simulink model "OberverForPMSM"  (R2018b)
settings: Solver=FixedStepAuto  StartTime=0.0  StopTime=inf  FixedStep=Ts  MaxStep=Ts  RelTol=1e-3  EnableMultiTasking=on
PreLoadFcn:
  | Ts=1e-6;
  | deci=20;
InitFcn:
  | Ts=5e-6;
  | deci=20;
undefined symbols (not defined in the file or in its folder): DiscIntNeverNeededParam, level
libraries: powerlib_extras x37, powerlib x18, powerlib_meascontrol x8, simulink x5, simulink_extras x4
(part 1 of 2)
Description:
  | Copyright 2013-2015 Ruan Jiayang, Tsinghua Univ.
settings Model: SimulationMode=accelerator  Creator=XiaoLei  LastModifiedBy=Administrator
settings SolverCC: AlgebraicLoopSolver=LineSearch  AutoInsertRateTranBlk=on
settings DataIOCC: InitialState=xInit  LimitDataPoints=on  SaveFinalState=on  SaveFormat=StructureWithTime  SignalLoggingSaveFormat=ModelDataLogs  SaveOutput=off  SignalLogging=off  SaveTime=off
settings OptimizationCC: ExpressionDepthLimit=2147483647  InitFltsAndDblsToZero=on  LifeSpan=inf
settings DebuggingCC: SaveWithParameterizedLinksMsg=none  UnderspecifiedInitializationDetection=Classic  MergeDetectMultiDrivingBlocksExec=none  SignalResolutionControl=TryResolveAllWithWarning  SolverPrmCheckMsg=warning  MultiTaskDSMMsg=warning  MultiTaskCondExecSysMsg=none  FcnCallInpInsideContextMsg=warning  UnconnectedInputMsg=none  UnconnectedOutputMsg=none  UnconnectedLineMsg=none  StateNameClashWarn=warning  SFUnexpectedBacktrackingDiag=warning  SFNoUnconditionalDefaultTransitionDiag=warning  SFExecutionAtInitializationDiag=none
settings HardwareCC: ProdBitPerPointer=32  ProdBitPerSizeT=32  ProdBitPerPtrDiffT=32  ProdLargestAtomicFloat=None  ProdIntDivRoundTo=Undefined  ProdEndianess=Unspecified  ProdWordSize=32  ProdHWDeviceType=32-bit Generic
settings ModelReferenceCC: PropagateSignalLabelsOutOfModel=off
settings SFSimCC: SimUseLocalCustomCode=off  SimParseCustomCode=off
settings RTWCC: RTWUseLocalCustomCode=off
settings CodeAppCC: StateflowObjectComments=on
settings GRTTargetCC: TargetFcnLib=ansi_tfl_tmw.mat  TargetLangStandard=C89/C90 (ANSI)  GeneratePreprocessorConditionals=Disable all  CombineOutputUpdateFcns=off  GRTInterface=on
settings ConfigComp: CovMetricSettings=dw  CovHtmlReporting=on  CovSaveCumulativeToWorkspaceVar=on  CovSaveSingleToWorkspaceVar=on  CovExternalEMLEnable=off

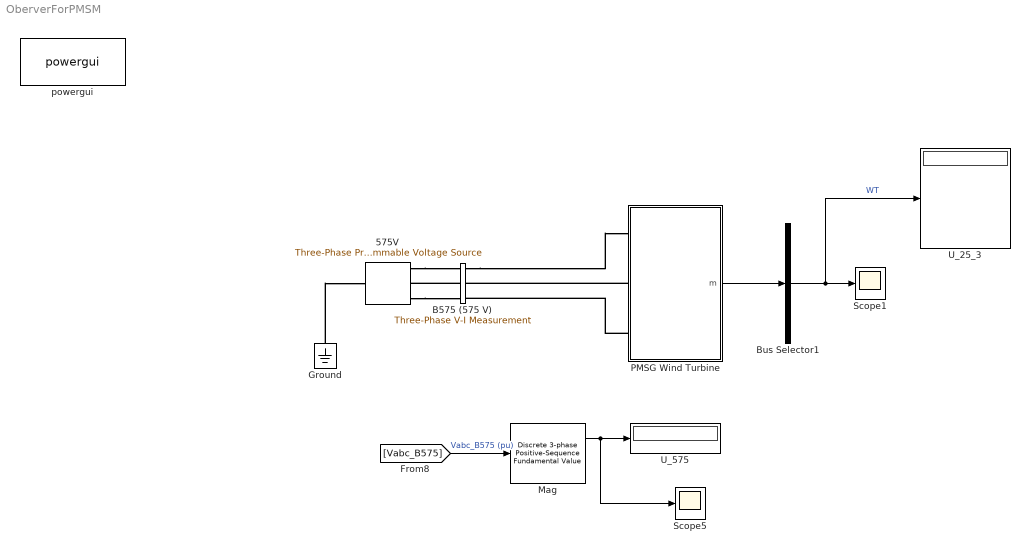
== system OberverForPMSM ==
  575V : powerlib/Electrical Sources/Three-Phase Programmable Voltage Source  PositiveSequence=[575 0 60]  VariationEntity=Amplitude  VariationType=Table of time-amplitude pairs  VariationTypeAlt=Step  VariationStep=-0.2  VariationRate=10  VariationMagnitude=0.3  VariationFrequency=2  VariationTiming=[0.05 0.05+5/60]  VariationPhaseA=off  Amplitudes=[1 0.5 1]  TimeValues=[0 20 20.3]  HarmonicGeneration=off  HarmonicA=[1 -0.1 0 2]  HarmonicB=[2 0.15 35 2]*0  Timing="[0.1  2]"  BusType=swing  Pref=0  Qref=0  Qmin=-inf  Qmax=inf
  B575 (575 V) : powerlib/Measurements/Three-Phase V-I Measurement  VoltageMeasurement=phase-to-ground  SetLabelV=on  LabelV=Vabc_B575  Vpu=on  VpuLL=off  CurrentMeasurement=yes  SetLabelI=on  LabelI=Iabc_B575  Ipu=on  Pbase=1.5e6  Vbase=575  OutputType=Complex  PhasorSimulation=off  PSBequivalent=0
  Bus Selector1 : BusSelector  OutputSignals=wr,Tem,Tm,PQ.P_pu,PQ.Q_pu  OutputAsBus=on
  Ground : powerlib/Elements/Ground  LConnTagsString=a
  Mag : powerlib_extras/Discrete Measurements/Discrete 3-phase Positive-Sequence Fundamental Value  Freq=60  Par_Init=[0 0]  Ts=Ts
  PMSG Wind Turbine : Subsystem  mask{Nb_wt=100, Vnom=575, Pnom1=4e6, Fnom=60, RL_grid=[0.003 0.3], CDC_link1=10000e-6, Vdc_nom=1150, Np=48, Fb_time_const=0.005}
      mask prompts: Nb_wt "Number of wind turbines"; Vnom "Rated L-L Voltage(V)"; Pnom1 "Rated Power(VA)"; Fnom "Rated Frequency(Hz)"; RL_grid "Grid-side coupling impedance(p.u.)"; CDC_link1 "DC bus capitance (F)"; Vdc_nom "DC capacitor voltage(V)"; Np "Number of pole pairs"; Fb_time_const "Feed back time constant(s)"
      mask init:
      | R_RL=RL_grid(1);
      | L_RL=RL_grid(2);
      | CDC_link=CDC_link1*Nb_wt;
      | Pnom=Pnom1*Nb_wt;
      | Inom=Pnom/sqrt(3)/Vnom;
      | Znom=Vnom/sqrt(3)/Inom;
      | Lnom=Znom/2/pi/Fnom;
      | Flux_nom=sqrt(2/3)*Vnom/2/pi/Fnom;
      | Rs_pu=0.027;
      | Ldq_pu=0.5131;
      | Rs=Rs_pu*Znom;
      | Ldq=Ldq_pu*Lnom;
      | Flux_pu=1.18842;
      | H=0.685+4.32;
      | J=(2*pi*Fnom/Np)^(-2)*2*H*Pnom;
      | Flux=Flux_pu*Flux_nom;
      | Vw_rated=12.1;
      | Wr_rated=1.1;
      | Radius=sqrt(Pnom1*2/1.12/pi/0.44/Vw_rated^3); %1.12 is the air density, 0.44 is the maximum wind conversion rate
      | Kratio=10.5*Vw_rated/Radius/Wr_rated; %10.5 is the optimal  tip speed ratio
  Scope1 : Scope
  Scope5 : Scope
  U_25_3 : Display
      settings: Decimation=round(0.1/Ts)
  U_575 : Display
      settings: Decimation=round(0.1/Ts)
  powergui : powerlib/powergui  SimulationMode=Discrete  SampleTime=Ts  frequency=50  Iterations=50  frequencyindice=0  Pbase=100e6  ErrMax=1e-4  UnitsV=kV  UnitsW=MW  buscounter=0  FunctionMessages=off  echomessages=off  EnableUseOfTLC=off  CurrentSourceSwitches=off  DisableSnubberDevices=off  DisableRonSwitches=off  DisableVfSwitches=off  DisplayEquations=off  SolverType=Tustin/Backward Euler (TBE)  Interpol=off  ExternalGateDelay=off  methode=off  Ts=100  x0status=blocks  SPID=off  SwTol=0  HookPort=off  RestoreLinks=warning  ResistiveCurrentMeasurement=off  Frange=[0:2:500]  Ylog=off  Xlog=on  ShowGrid=off  save=off  variable=ZData  structure=0  ZoomFFT=on  StartTime=0.0  cycles=1  DisplayStyle=1  fundamental=60  FreqAxis=off  MaxFrequency=1000  frequencyindicesteady=1  RmsSteady=1  display=off
  wires:
  [Vabc_B575] -> Mag/1  "Vabc_B575 (pu)"
  Mag/1 -> U_575/1, Scope5/1
  Bus Selector1/1 -> U_25_3/1, Scope1/1  "WT"
  PMSG Wind Turbine/1(m) -> Bus Selector1/1
  connections:
  Ground/LConn1 -- 575V/LConn1
  B575 (575 V)/LConn2 -- 575V/RConn2
  575V/RConn1 -- B575 (575 V)/LConn1
  575V/RConn3 -- B575 (575 V)/LConn3
  B575 (575 V)/RConn1 -- PMSG Wind Turbine/LConn1
  PMSG Wind Turbine/LConn2 -- B575 (575 V)/RConn2
  PMSG Wind Turbine/LConn3 -- B575 (575 V)/RConn3

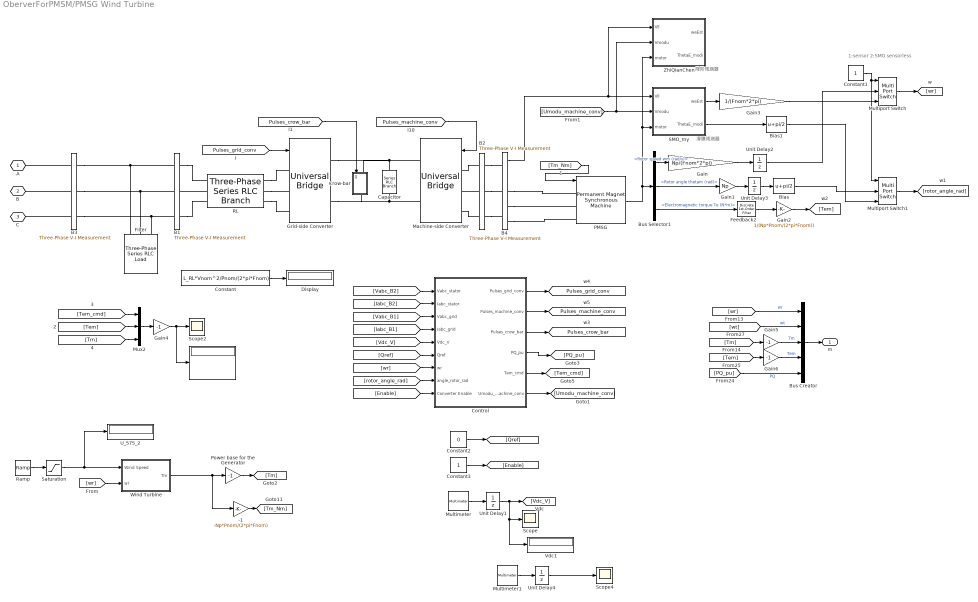
== system OberverForPMSM/PMSG Wind Turbine ==
  note: 滑膜观测器
  note: 1:sensor
      | 2:SMO sensorless
  note: 降阶观测器
  "                                       " : Display
      settings: Decimation=round(0.1/Ts)
  -1 : Gain  Gain=-Np*Pnom/(2*pi*Fnom)
  B1 : powerlib/Measurements/Three-Phase V-I Measurement  VoltageMeasurement=phase-to-ground  SetLabelV=on  LabelV=Vabc_B1  Vpu=on  VpuLL=off  CurrentMeasurement=yes  SetLabelI=on  LabelI=Iabc_B1  Ipu=on  Pbase=Pnom  Vbase=Vnom  OutputType=Complex  PhasorSimulation=off  PSBequivalent=0
  B2 : powerlib/Measurements/Three-Phase V-I Measurement  VoltageMeasurement=phase-to-ground  SetLabelV=on  LabelV=Vabc_B2  Vpu=on  VpuLL=off  CurrentMeasurement=yes  SetLabelI=on  LabelI=Iabc_B2  Ipu=on  Pbase=Pnom  Vbase=Vnom  OutputType=Complex  PhasorSimulation=off  PSBequivalent=0
  B3 : powerlib/Measurements/Three-Phase V-I Measurement  VoltageMeasurement=phase-to-ground  SetLabelV=on  LabelV=Vabc_B0  Vpu=on  VpuLL=off  CurrentMeasurement=yes  SetLabelI=on  LabelI=Iabc_B0  Ipu=on  Pbase=Pnom  Vbase=Vnom  OutputType=Complex  PhasorSimulation=off  PSBequivalent=0
  B4 : powerlib/Measurements/Three-Phase V-I Measurement  VoltageMeasurement=phase-to-phase  SetLabelV=off  LabelV=Vabc_WWW  Vpu=off  VpuLL=off  CurrentMeasurement=yes  SetLabelI=off  LabelI=Iabc_B2  Ipu=off  Pbase=Pnom  Vbase=Vnom  OutputType=Complex  PhasorSimulation=off  PSBequivalent=0
  Bias : Bias  Bias=pi/2
  Bias1 : Bias  Bias=pi/2
  Bus Creator : BusCreator  Inputs=5
  Bus Selector1 : BusSelector  OutputSignals=Rotor speed wm (rad/s),Rotor angle thetam (rad),Electromagnetic torque Te (N*m)
  Capacitor : powerlib/Elements/Series RLC Branch  LConnTagsString=__new0  RConnTagsString=__new0  BranchType=C  Resistance=1e-5  Inductance=1e-3  SetiL0=off  InitialCurrent=0  Capacitance=CDC_link  Setx0=on  InitialVoltage=Vdc_nom  Measurements=Branch voltage
  Constant : Constant  Value=L_RL*Vnom^2/Pnom/(2*pi*Fnom)
  Constant1 : Constant
  Constant2 : Constant  Value=0  SampleTime=Ts
  Constant3 : Constant  SampleTime=Ts
  Control : Subsystem
  Crow-bar : Subsystem
  Display : Display
  Feedback2 : powerlib_extras/Discrete  Control Blocks/Discrete 1st-Order Filter  FilterType=Lowpass  Tc=0.02  Ts=Ts  Initialize=on  Vac_Init=[0 -25 60]  Vdc_Init=0  PlotResponse=off  param1=[1 500 0.1]
  Filter : powerlib/Elements/Three-Phase Series RLC Load  LConnTagsString=A|B|C  Configuration=Y (grounded)  NominalVoltage=Vnom  Vabc=[1e3 1e3 1e3]  Vabcp=[1e3 1e3 1e3]  NominalFrequency=Fnom  UnbalancedPower=off  ActivePower=120e3/50*Nb_wt  InductivePower=0  CapacitivePower=120e3*Nb_wt  Pabc=[10e3 9e3 11e3]  QLabc=[100 90 110]  QCabc=[100 90 110]  Pabcp=[10e3 9e3 11e3]  QLabcp=[100 90 110]  QCabcp=[100 90 110]  Measurements=None  LoadType=constant Z
  Gain : Gain  Gain=Np/(Fnom*2*pi)
  Gain1 : Gain  Gain=Np
  Gain2 : Gain  Gain=1/(Np*Pnom/(2*pi*Fnom))
  Gain3 : Gain  Gain=1/(Fnom*2*pi)
  Gain4 : Gain  Gain=-1
  Gain5 : Gain  Gain=-1
  Gain6 : Gain  Gain=-1
  Grid-side Converter : powerlib/Power Electronics/Universal Bridge  Arms=3  SnubberResistance=1e5/Nb_wt  SnubberCapacitance=inf  Device=IGBT / Diodes  Ron=1e-5/Nb_wt  Lon=0  ForwardVoltages="[  0  0  ]"  ForwardVoltage=0  GTOparameters=[ 10e-6 , 20e-6 ]  IGBTparameters=[0 , 0]  Measurements=None  Measurements_2=None  converterType=Rectifier
  Machine-side Converter : powerlib/Power Electronics/Universal Bridge  Arms=3  SnubberResistance=1e5/Nb_wt  SnubberCapacitance=inf  Device=IGBT / Diodes  Ron=1e-5/Nb_wt  Lon=0  ForwardVoltages="[  0  0  ]"  ForwardVoltage=0  GTOparameters=[ 10e-6 , 20e-6 ]  IGBTparameters=[0 , 0]  Measurements=None  Measurements_2=None  converterType=Rectifier
  Multimeter : powerlib/Measurements/Multimeter  PhasorSimulation=off  OutputType=Complex  sel=1  L=2  Gain=1  yselected={'Ub: PMSG Wind Turbine/Capacitor'};  PSBOutputType=1  PSBequivalent=0  AxesSetting=[0,0.1,-100,100]  Display=0  SavedBlockNames=-11
  Multimeter1 : powerlib/Measurements/Multimeter  PhasorSimulation=off  OutputType=Complex  sel=2  L=2  Gain=1  yselected={'Ib: PMSG Wind Turbine/Crow-bar/R'};  PSBOutputType=1  PSBequivalent=0  AxesSetting=[0,0.1,-100,100]  Display=0  SavedBlockNames=-11
  Multiport Switch : MultiPortSwitch  Inputs=2
  Multiport Switch1 : MultiPortSwitch  Inputs=2
  Mux2 : Mux  Inputs=3
  PMSG : powerlib/Machines/Permanent Magnet Synchronous Machine  NbPhases=3  FluxDistribution=Sinusoidal  RotorType=Salient-pole  MechanicalLoad=Torque Tm  PresetModel=No  ShowDetailedParameters=on  MeasurementBus=off  Resistance=Rs  Inductance=8.5e-3  dqInductances="[Ldq  Ldq]"  La=0.000395  MachineConstant=Flux linkage established by magnets (V.s)  Flux=Flux  VoltageCst=12885.2109  TorqueCst=106.5598  Flat=120  Mechanical=[J 0*Nb_wt Np]  PolePairs=Np  InitialConditions=[(2*pi*Fnom/Np)*1,0, 0,0]  InitialConditions5ph=[0 0 0 0 0 0]  TsPowergui=0  TsBlock=Ts  RefAngle=90 degrees behind phase A axis (modified Park)
      settings: SourceProductName=Simscape Power Systems
  Power base for the Generator : Gain  Gain=-1  SaturateOnIntegerOverflow=on  OutDataTypeStr=Inherit: Same as input  ParamDataTypeStr=Inherit: Same as input
  RL : powerlib/Elements/Three-Phase Series RLC Branch  LConnTagsString=A|B|C  RConnTagsString=A|B|C  BranchType=RL  Resistance=R_RL*Vnom^2/Pnom  Inductance=L_RL*Vnom^2/Pnom/(2*pi*Fnom)  Capacitance=1.0  Measurements=None
  Ramp : simulink/Sources/Ramp  slope=1  start=5  InitialOutput=10
  SMO_my : Subsystem
  Saturation : Saturate  UpperLimit=12  LowerLimit=7
  Scope : Scope
  Scope2 : Scope
  Scope4 : Scope
  U_575_2 : Display
      settings: Decimation=round(0.1/Ts)
  Unit Delay{1..4} (4 alike) : UnitDelay  SampleTime=Ts
  Vdc1 : Display
      settings: Decimation=round(0.1/Ts)
  Wind Turbine : Subsystem
  ZhiQianChen : Subsystem
  A : PMIOPort  Tag=PMCPort  Side=Left
  B : PMIOPort  Tag=PMCPort  Port=2  Side=Left
  C : PMIOPort  Tag=PMCPort  Port=3  Side=Left
  m : Outport
  tag scope: Pulses_crow_bar=global, Pulses_grid_conv=global, Pulses_machine_conv=global
  wires:
  Unit Delay1/1 -> [Vdc_V], Scope/1, Vdc1/1
  PMSG/1 -> ZhiQianChen/3(motor), SMO_my/3(motor), Bus Selector1/1
  Bus Selector1/1 -> Gain/1  "<Rotor speed wm (rad/s)>"
  Gain/1 -> Unit Delay2/1
  Gain1/1 -> Unit Delay3/1
  Bus Selector1/2 -> Gain1/1  "<Rotor angle thetam (rad)>"
  [Qref] -> Control/6(Qref)
  [Vdc_V] -> Control/5(Vdc_V)
  [Iabc_B1] -> Control/4(Iabc_grid)
  [Vabc_B1] -> Control/3(Vabc_grid)
  [Vabc_B2] -> Control/1(Vabc_stator)
  [Iabc_B2] -> Control/2(Iabc_stator)
  [Enable] -> Control/9(Converter Enable)
  Constant3/1 -> [Enable]
  Constant2/1 -> [Qref]
  [Pulses_grid_conv] -> Grid-side Converter/1
  [Pulses_machine_conv] -> Machine-side Converter/1
  Control/1(Pulses_grid_conv) -> [Pulses_grid_conv]
  Control/2(Pulses_machine_conv) -> [Pulses_machine_conv]
  [wr] -> Control/7(wr)
  [rotor_angle_rad] -> Control/8(angle_rotor_rad)
  Unit Delay3/1 -> Bias/1
  [Tm_Nm] -> PMSG/1
  Gain2/1 -> [Tem]
  Control/5(Tem_cmd) -> [Tem_cmd]
  [Tem] -> Mux2/2
  [Tem_cmd] -> Mux2/1
  [Tm] -> Mux2/3
  Mux2/1 -> Gain4/1
  Gain4/1 -> Scope2/1, "                                       "/1
  Multimeter/1 -> Unit Delay1/1
  Control/3(Pulses_crow_bar) -> [Pulses_crow_bar]
  Unit Delay4/1 -> Scope4/1
  Multimeter1/1 -> Unit Delay4/1
  [Pulses_crow_bar] -> Crow-bar/1(g)
  Bus Creator/1 -> m/1
  [Tm] -> Gain5/1
  [Tem] -> Gain6/1
  [wr] -> Bus Creator/1  "wr"
  [wt] -> Bus Creator/2  "wt"
  Gain5/1 -> Bus Creator/3  "Tm"
  Gain6/1 -> Bus Creator/4  "Tem"
  [PQ_pu] -> Bus Creator/5  "PQ"
  Wind Turbine/1(Tm) -> Power base for the Generator/1, -1/1
  Power base for the Generator/1 -> [Tm]
  -1/1 -> [Tm_Nm]
  Ramp/1 -> Saturation/1
  Control/4(PQ_pu) -> [PQ_pu]
  Saturation/1 -> Wind Turbine/1(Wind Speed), U_575_2/1
  [wr] -> Wind Turbine/2(wr)
  Feedback2/1 -> Gain2/1
  Bus Selector1/3 -> Feedback2/1  "<Electromagnetic torque Te (N*m)>"
  B4/1 -> ZhiQianChen/1(Vll), SMO_my/1(Vll)
  Constant/1 -> Display/1
  Control/6(Umodu_machine_conv) -> [Umodu_machine_conv]
  [Umodu_machine_conv] -> ZhiQianChen/2(Vmodu), SMO_my/2(Vmodu)
  SMO_my/1(weEst) -> Gain3/1
  SMO_my/2(ThetaE_modi) -> Bias1/1
  Multiport Switch/1 -> [wr]
  Unit Delay2/1 -> Multiport Switch/2
  Bias/1 -> Multiport Switch1/2
  Constant1/1 -> Multiport Switch1/1, Multiport Switch/1
  Multiport Switch1/1 -> [rotor_angle_rad]
  Gain3/1 -> Multiport Switch/3
  Bias1/1 -> Multiport Switch1/3
  connections:
  RL/RConn1 -- Grid-side Converter/LConn1
  RL/RConn2 -- Grid-side Converter/LConn2
  RL/RConn3 -- Grid-side Converter/LConn3
  Filter/LConn1 -- B1/LConn1 -- B3/RConn1
  Filter/LConn2 -- B1/LConn2 -- B3/RConn2
  Filter/LConn3 -- B1/LConn3 -- B3/RConn3
  B1/RConn1 -- RL/LConn1
  RL/LConn2 -- B1/RConn2
  B1/RConn3 -- RL/LConn3
  B2/LConn1 -- Machine-side Converter/LConn1
  Machine-side Converter/LConn3 -- B2/LConn3
  B2/LConn2 -- Machine-side Converter/LConn2
  Grid-side Converter/RConn1 -- Crow-bar/LConn1 -- Machine-side Converter/RConn1 -- Capacitor/LConn1
  Grid-side Converter/RConn2 -- Crow-bar/RConn1 -- Machine-side Converter/RConn2 -- Capacitor/RConn1
  B3/LConn1 -- A/RConn1
  B3/LConn2 -- B/RConn1
  B3/LConn3 -- C/RConn1
  B2/RConn1 -- B4/LConn1
  B2/RConn2 -- B4/LConn2
  B2/RConn3 -- B4/LConn3
  B4/RConn1 -- PMSG/LConn1
  B4/RConn2 -- PMSG/LConn2
  B4/RConn3 -- PMSG/LConn3

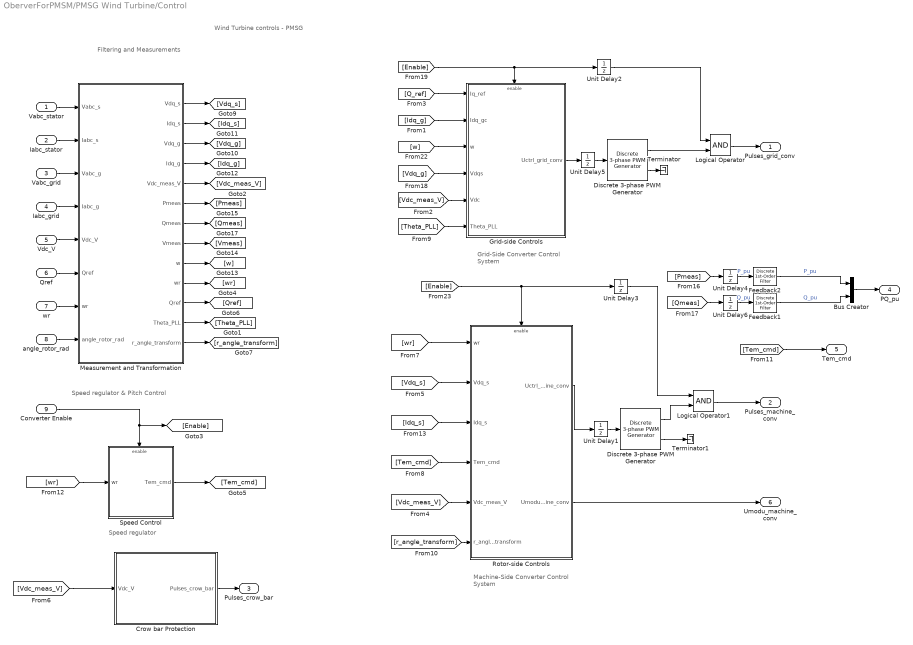
== system OberverForPMSM/PMSG Wind Turbine/Control ==
  note: Wind Turbine controls - PMSG
  note: Filtering and
      | Measurements
  note: Speed regulator & Pitch Control
  note: Speed regulator
  note: Machine-Side Converter
      | Control System
  note: Grid-Side Converter
      | Control System
  Vabc_stator : Inport
  Iabc_stator : Inport  Port=2
  Vabc_grid : Inport  Port=3
  Iabc_grid : Inport  Port=4
  Vdc_V : Inport  Port=5
  Qref : Inport  Port=6
  wr : Inport  Port=7
  angle_rotor_rad : Inport  Port=8
  Converter Enable : Inport  Port=9
  Bus Creator : BusCreator  Inputs=2
  Crow bar Protection : Subsystem
  Discrete 3-phase PWM Generator : powerlib_extras/Discrete  Control Blocks/Discrete 3-phase PWM Generator  ModulatorType=2-level  ModulatorMode=Un-synchronized  nF=27  Fc=2700  ModulatingSignals=off  m=0.2  Freq=60  Phase=0  Ts=Ts
  "Discrete 3-phase PWM Generator " : powerlib_extras/Discrete  Control Blocks/Discrete 3-phase PWM Generator  ModulatorType=2-level  ModulatorMode=Un-synchronized  nF=27  Fc=1620  ModulatingSignals=off  m=0.2  Freq=60  Phase=0  Ts=Ts
  Feedback1 : powerlib_extras/Discrete  Control Blocks/Discrete 1st-Order Filter  FilterType=Lowpass  Tc=0.01  Ts=Ts  Initialize=on  Vac_Init=[0 -25 60]  Vdc_Init=0  PlotResponse=off  param1=[1 500 0.1]
  Feedback2 : powerlib_extras/Discrete  Control Blocks/Discrete 1st-Order Filter  FilterType=Lowpass  Tc=0.01  Ts=Ts  Initialize=on  Vac_Init=[0 -25 60]  Vdc_Init=0  PlotResponse=off  param1=[1 500 0.1]
  Grid-side Controls : Subsystem
  Logical Operator : Logic  AllPortsSameDT=off  OutDataTypeStr=boolean
  Logical Operator1 : Logic  AllPortsSameDT=off  OutDataTypeStr=boolean
  Measurement and Transformation : Subsystem
  Rotor-side Controls : Subsystem
  Speed Control : Subsystem
  Terminator : Terminator
  Terminator1 : Terminator
  Unit Delay{1..6} (6 alike) : UnitDelay  SampleTime=Ts
  Pulses_grid_conv : Outport
  Pulses_machine_conv : Outport  Port=2
  Pulses_crow_bar : Outport  Port=3
  PQ_pu : Outport  Port=4
  Tem_cmd : Outport  Port=5
  Umodu_machine_conv : Outport  Port=6
  wires:
  [Pmeas] -> Unit Delay4/1
  [Qmeas] -> Unit Delay6/1
  wr/1 -> Measurement and Transformation/7(wr)
  Qref/1 -> Measurement and Transformation/6(Qref)
  Vdc_V/1 -> Measurement and Transformation/5(Vdc_V)
  Measurement and Transformation/11("Qref ") -> [Qref]
  Measurement and Transformation/10("wr ") -> [wr]
  Measurement and Transformation/5(Vdc_meas_V) -> [Vdc_meas_V]
  Measurement and Transformation/9(w) -> [w]
  Measurement and Transformation/6(Pmeas) -> [Pmeas]
  Measurement and Transformation/4(Idq_g) -> [Idq_g]
  Measurement and Transformation/3(Vdq_g) -> [Vdq_g]
  Measurement and Transformation/2(Idq_s) -> [Idq_s]
  angle_rotor_rad/1 -> Measurement and Transformation/8(angle_rotor_rad)
  Iabc_stator/1 -> Measurement and Transformation/2(Iabc_s)
  Iabc_grid/1 -> Measurement and Transformation/4(Iabc_g)
  Vabc_grid/1 -> Measurement and Transformation/3(Vabc_g)
  Vabc_stator/1 -> Measurement and Transformation/1(Vabc_s)
  Measurement and Transformation/7(Qmeas) -> [Qmeas]
  Measurement and Transformation/8(Vmeas) -> [Vmeas]
  Measurement and Transformation/12(Theta_PLL) -> [Theta_PLL]
  Measurement and Transformation/13(r_angle_transform) -> [r_angle_transform]
  Speed Control/1(Tem_cmd) -> [Tem_cmd]
  [wr] -> Speed Control/1(wr)
  Converter Enable/1 -> Speed Control/Enable, [Enable]
  [Tem_cmd] -> Tem_cmd/1
  Measurement and Transformation/1(Vdq_s) -> [Vdq_s]
  Grid-side Controls/1(Uctrl_grid_conv) -> Unit Delay5/1
  Discrete 3-phase PWM Generator/2 -> Terminator/1
  Unit Delay5/1 -> Discrete 3-phase PWM Generator/1
  [Vdc_meas_V] -> Grid-side Controls/5(Vdc)
  [Vdq_g] -> Grid-side Controls/4(Vdqs)
  [w] -> Grid-side Controls/3(w)
  [Idq_g] -> Grid-side Controls/2(Idq_gc)
  [Q_ref] -> Grid-side Controls/1(Iq_ref)
  [Theta_PLL] -> Grid-side Controls/6(Theta_PLL)
  [Enable] -> Grid-side Controls/Enable, Unit Delay2/1
  Logical Operator/1 -> Pulses_grid_conv/1
  Discrete 3-phase PWM Generator/1 -> Logical Operator/2
  Unit Delay2/1 -> Logical Operator/1
  "Discrete 3-phase PWM Generator "/2 -> Terminator1/1
  Unit Delay1/1 -> "Discrete 3-phase PWM Generator "/1
  [Enable] -> Unit Delay3/1, Rotor-side Controls/Enable
  Logical Operator1/1 -> Pulses_machine_conv/1
  "Discrete 3-phase PWM Generator "/1 -> Logical Operator1/2
  Unit Delay3/1 -> Logical Operator1/1
  [wr] -> Rotor-side Controls/1(wr)
  [Vdc_meas_V] -> Rotor-side Controls/5(Vdc_meas_V)
  [r_angle_transform] -> Rotor-side Controls/6(r_angle_transform)
  [Vdq_s] -> Rotor-side Controls/2(" Vdq_s")
  [Idq_s] -> Rotor-side Controls/3(Idq_s)
  Rotor-side Controls/1(Uctrl_machine_conv) -> Unit Delay1/1
  [Tem_cmd] -> Rotor-side Controls/4(Tem_cmd)
  Unit Delay4/1 -> Feedback2/1  "P_pu"
  Feedback2/1 -> Bus Creator/1  "P_pu"
  Unit Delay6/1 -> Feedback1/1  "Q_pu"
  Feedback1/1 -> Bus Creator/2  "Q_pu"
  Crow bar Protection/1(Pulses_crow_bar) -> Pulses_crow_bar/1
  [Vdc_meas_V] -> Crow bar Protection/1(Vdc_V)
  Bus Creator/1 -> PQ_pu/1
  Rotor-side Controls/2(Umodu_machine_conv) -> Umodu_machine_conv/1

== system OberverForPMSM/PMSG Wind Turbine/Crow-bar ==
  g : Inport
  IGBT : powerlib/Power Electronics/IGBT//Diode  Ron=1e-5/Nb_wt  Rs=1e5/Nb_wt  Cs=inf  Measurements=off
  R : powerlib/Elements/Series RLC Branch  LConnTagsString=__new0  RConnTagsString=__new0  BranchType=R  Resistance=1/Nb_wt  Inductance=1e-3  SetiL0=off  InitialCurrent=0  Capacitance=1e-6  Setx0=off  InitialVoltage=0  Measurements=Branch current
  + : PMIOPort  Side=Left
  - : PMIOPort  Port=2  Side=Right
  wires:
  g/1 -> IGBT/1
  connections:
  R/LConn1 -- IGBT/RConn1
  +/RConn1 -- IGBT/LConn1
  -/RConn1 -- R/RConn1

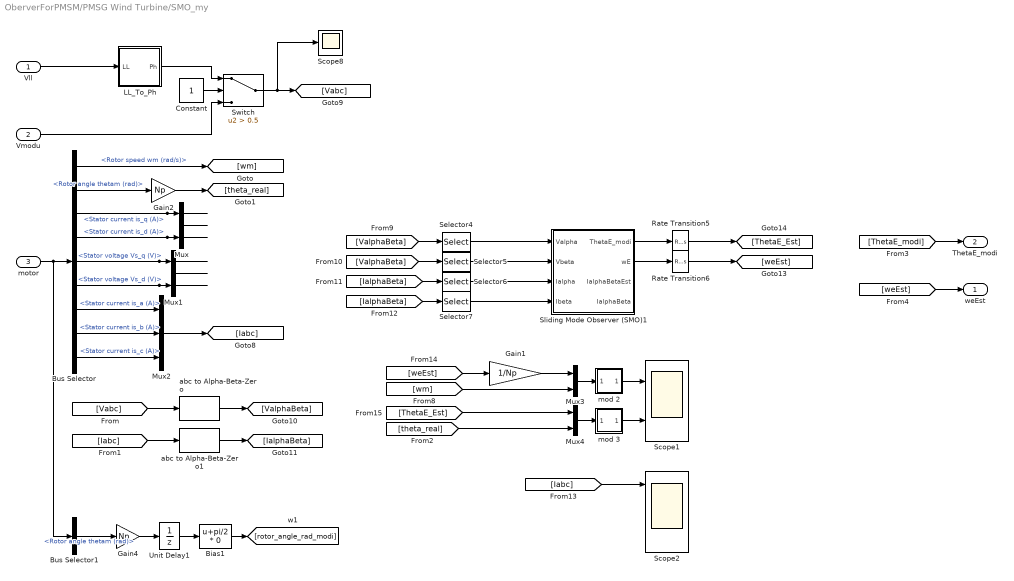
== system OberverForPMSM/PMSG Wind Turbine/SMO_my ==
  Vll : Inport
  Vmodu : Inport  Port=2
  motor : Inport  Port=3
  Bias1 : Bias  Bias=pi/2 * 0
  Bus Selector : BusSelector  OutputSignals=Rotor speed wm (rad/s),Rotor angle thetam (rad),Stator current is_q (A),Stator current is_d (A),Stator voltage Vs_q (V),Stator voltage Vs_d (V),Stator current is_a (A),Stator current is_b (A),Stator current is_c (A)
  Bus Selector1 : BusSelector  OutputSignals=Rotor angle thetam (rad)
  Constant : Constant
  Gain1 : Gain  Gain=1/Np
  Gain2 : Gain  Gain=Np
  Gain4 : Gain  Gain=Np
  LL_To_Ph : Subsystem
  Mux{,1,3..4} (4 alike) : Mux  Inputs=2
  Mux2 : Mux  Inputs=3
  Rate Transition5 : RateTransition
  Rate Transition6 : RateTransition
  Scope1 : Scope  NumInputPorts=2
  Scope2 : Scope  NumInputPorts=3
  Scope8 : Scope
  Selector4 : Selector  InputPortWidth=3  IndexOptions=Index vector (dialog)  Indices=[1]  OutputSizes=1
  Selector5 : Selector  InputPortWidth=3  IndexOptions=Index vector (dialog)  Indices=[2]  OutputSizes=1
  Selector6 : Selector  InputPortWidth=3  IndexOptions=Index vector (dialog)  Indices=[1]  OutputSizes=1
  Selector7 : Selector  InputPortWidth=3  IndexOptions=Index vector (dialog)  Indices=[2]  OutputSizes=1
  Sliding Mode Observer (SMO)1 : Subsystem  mask(dummy){Tctl=1/100e3}
      mask help: dummy
  Switch : Switch  Criteria=u2 > Threshold  Threshold=0.5
  Unit Delay1 : UnitDelay  SampleTime=Ts
  abc to Alpha-Beta-Zero : powerlib_meascontrol/Transformations/abc to Alpha-Beta-Zero
      settings: SourceProductName=Simscape Power Systems
  abc to Alpha-Beta-Zero1 : powerlib_meascontrol/Transformations/abc to Alpha-Beta-Zero
      settings: SourceProductName=Simscape Power Systems
  mod 2 : Subsystem
  mod 3 : Subsystem
  weEst : Outport
  ThetaE_modi : Outport  Port=2
  wires:
  motor/1 -> Bus Selector1/1, Bus Selector/1
  Bus Selector/1 -> [wm]  "<Rotor speed wm (rad/s)>"
  Bus Selector/2 -> Gain2/1  "<Rotor angle thetam (rad)>"
  Bus Selector/4 -> Mux/2  "<Stator current is_d (A)>"
  Bus Selector/3 -> Mux/1  "<Stator current is_q (A)>"
  Mux/1 -> ?
  Mux1/1 -> ?
  Bus Selector/5 -> Mux1/1  "<Stator voltage Vs_q (V)>"
  Bus Selector/6 -> Mux1/2  "<Stator voltage Vs_d (V)>"
  Bus Selector/7 -> Mux2/1  "<Stator current is_a (A)>"
  Bus Selector/8 -> Mux2/2  "<Stator current is_b (A)>"
  Bus Selector/9 -> Mux2/3  "<Stator current is_c (A)>"
  Mux2/1 -> [Iabc]
  Vll/1 -> LL_To_Ph/1(LL)
  [Vabc] -> abc to Alpha-Beta-Zero/1
  [Iabc] -> abc to Alpha-Beta-Zero1/1
  abc to Alpha-Beta-Zero/1 -> [ValphaBeta]
  [ValphaBeta] -> Selector4/1
  [ValphaBeta] -> Selector5/1
  [IalphaBeta] -> Selector7/1
  [IalphaBeta] -> Selector6/1
  [Iabc] -> Scope2/1
  Selector4/1 -> Sliding Mode Observer (SMO)1/1(Valpha)
  Selector5/1 -> Sliding Mode Observer (SMO)1/2(Vbeta)
  Selector6/1 -> Sliding Mode Observer (SMO)1/3(Ialpha)
  Selector7/1 -> Sliding Mode Observer (SMO)1/4(Ibeta)
  Sliding Mode Observer (SMO)1/2(wE) -> Rate Transition6/1
  [weEst] -> Gain1/1
  Sliding Mode Observer (SMO)1/1(ThetaE_modi) -> Rate Transition5/1
  Mux3/1 -> mod 2/1(In1)
  mod 2/1(Out1) -> Scope1/1
  Mux4/1 -> mod 3/1(In1)
  mod 3/1(Out1) -> Scope1/2
  abc to Alpha-Beta-Zero1/1 -> [IalphaBeta]
  Switch/1 -> Scope8/1, [Vabc]
  Constant/1 -> Switch/2
  LL_To_Ph/1(Ph) -> Switch/1
  Vmodu/1 -> Switch/3
  Gain1/1 -> Mux3/1
  [wm] -> Mux3/2
  Rate Transition5/1 -> [ThetaE_Est]
  Rate Transition6/1 -> [weEst]
  Bias1/1 -> [rotor_angle_rad_modi]
  Unit Delay1/1 -> Bias1/1
  Gain4/1 -> Unit Delay1/1
  Bus Selector1/1 -> Gain4/1  "<Rotor angle thetam (rad)>"
  [ThetaE_modi] -> ThetaE_modi/1
  [weEst] -> weEst/1
  [ThetaE_Est] -> Mux4/1
  [theta_real] -> Mux4/2
  Gain2/1 -> [theta_real]

== system OberverForPMSM/PMSG Wind Turbine/Wind Turbine ==
  Wind Speed : Inport
  wr : Inport  Port=2
  Constant1 : Constant  Value=1.0*1.2  SampleTime=Ts
  Display1 : Display
      settings: Decimation=round(0.1/Ts)
  Turbine Rotor : Subsystem
  pitch angle controller : Subsystem
  Tm : Outport
  wires:
  Turbine Rotor/1(Tm) -> Tm/1  "Tm"
  Constant1/1 -> pitch angle controller/2(Ref)
  pitch angle controller/1(pitch) -> Display1/1, Turbine Rotor/3(pitch)
  Wind Speed/1 -> Turbine Rotor/1(u)
  wr/1 -> pitch angle controller/1(wg), Turbine Rotor/2(wr)

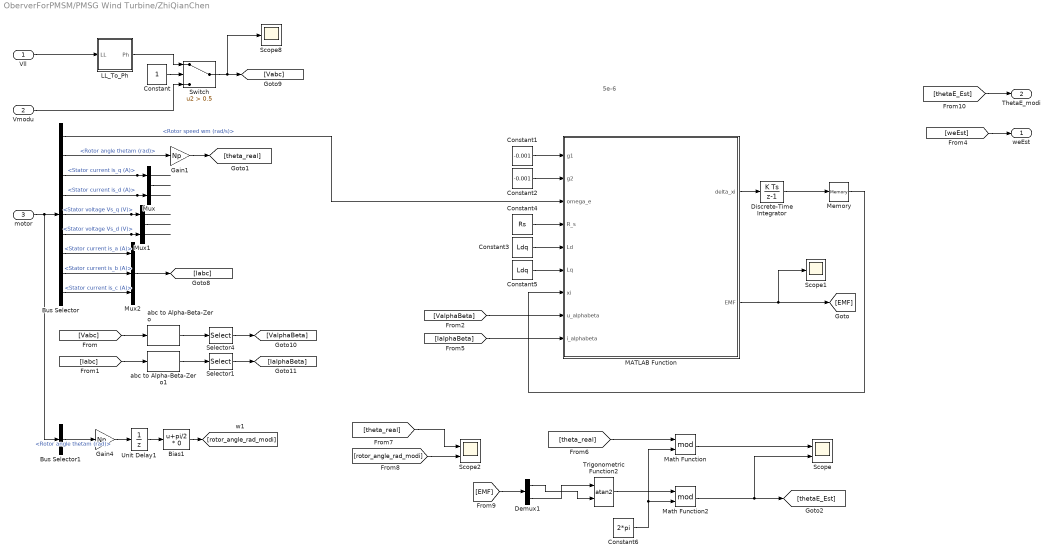
== system OberverForPMSM/PMSG Wind Turbine/ZhiQianChen ==
  note: 5e-6
  Vll : Inport
  Vmodu : Inport  Port=2
  motor : Inport  Port=3
  Bias1 : Bias  Bias=pi/2 * 0
  Bus Selector : BusSelector  OutputSignals=Rotor speed wm (rad/s),Rotor angle thetam (rad),Stator current is_q (A),Stator current is_d (A),Stator voltage Vs_q (V),Stator voltage Vs_d (V),Stator current is_a (A),Stator current is_b (A),Stator current is_c (A)
  Bus Selector1 : BusSelector  OutputSignals=Rotor angle thetam (rad)
  Constant : Constant
  Constant1 : Constant  Value=-0.001
  Constant2 : Constant  Value=-0.001
  Constant3 : Constant  Value=Ldq
  Constant4 : Constant  Value=Rs
  Constant5 : Constant  Value=Ldq
  Constant6 : Constant  Value=2*pi
  Demux1 : Demux  Outputs=2
  Discrete-Time Integrator : DiscreteIntegrator  SampleTime=-1  ICPrevOutput=DiscIntNeverNeededParam  ICPrevScaledInput=DiscIntNeverNeededParam
  Gain1 : Gain  Gain=Np
  Gain4 : Gain  Gain=Np
  LL_To_Ph : Subsystem
  MATLAB Function : MATLAB Function  TreatAsAtomicUnit=on
  Math Function : Math  Operator=mod  SaturateOnIntegerOverflow=on
  Math Function2 : Math  Operator=mod  SaturateOnIntegerOverflow=on
  Memory : Memory
  Mux : Mux  Inputs=2
  Mux1 : Mux  Inputs=2
  Mux2 : Mux  Inputs=3
  Scope : Scope  NumInputPorts=2
  Scope1 : Scope
  Scope2 : Scope  NumInputPorts=2
  Scope8 : Scope
  Selector1 : Selector  InputPortWidth=3  IndexOptions=Index vector (dialog)  Indices=[1 2]  OutputSizes=1
  Selector4 : Selector  InputPortWidth=3  IndexOptions=Index vector (dialog)  Indices=[1 2]  OutputSizes=1
  Switch : Switch  Criteria=u2 > Threshold  Threshold=0.5
  Trigonometric Function2 : Trigonometry  Operator=atan2  ApproximationMethod=CORDIC
  Unit Delay1 : UnitDelay  SampleTime=Ts
  abc to Alpha-Beta-Zero : powerlib_meascontrol/Transformations/abc to Alpha-Beta-Zero
      settings: SourceProductName=Simscape Power Systems
  abc to Alpha-Beta-Zero1 : powerlib_meascontrol/Transformations/abc to Alpha-Beta-Zero
      settings: SourceProductName=Simscape Power Systems
  weEst : Outport
  ThetaE_modi : Outport  Port=2
  wires:
  [weEst] -> weEst/1
  [thetaE_Est] -> ThetaE_modi/1
  Bus Selector1/1 -> Gain4/1  "<Rotor angle thetam (rad)>"
  Gain4/1 -> Unit Delay1/1
  Unit Delay1/1 -> Bias1/1
  Bias1/1 -> [rotor_angle_rad_modi]
  Vmodu/1 -> Switch/3
  LL_To_Ph/1(Ph) -> Switch/1
  Constant/1 -> Switch/2
  Switch/1 -> [Vabc], Scope8/1
  [Iabc] -> abc to Alpha-Beta-Zero1/1
  [Vabc] -> abc to Alpha-Beta-Zero/1
  Vll/1 -> LL_To_Ph/1(LL)
  Mux2/1 -> [Iabc]
  Bus Selector/9 -> Mux2/3  "<Stator current is_c (A)>"
  Bus Selector/8 -> Mux2/2  "<Stator current is_b (A)>"
  Bus Selector/7 -> Mux2/1  "<Stator current is_a (A)>"
  Bus Selector/6 -> Mux1/2  "<Stator voltage Vs_d (V)>"
  Bus Selector/5 -> Mux1/1  "<Stator voltage Vs_q (V)>"
  Mux1/1 -> ?
  Mux/1 -> ?
  Bus Selector/3 -> Mux/1  "<Stator current is_q (A)>"
  Bus Selector/4 -> Mux/2  "<Stator current is_d (A)>"
  Bus Selector/2 -> Gain1/1  "<Rotor angle thetam (rad)>"
  Bus Selector/1 -> MATLAB Function/3(omega_e)  "<Rotor speed wm (rad/s)>"
  motor/1 -> Bus Selector/1, Bus Selector1/1
  Constant1/1 -> MATLAB Function/1(g1)
  Constant2/1 -> MATLAB Function/2(g2)
  Constant5/1 -> MATLAB Function/6(Lq)
  Constant3/1 -> MATLAB Function/5(Ld)
  Constant4/1 -> MATLAB Function/4(R_s)
  MATLAB Function/1(delta_xi) -> Discrete-Time Integrator/1
  Discrete-Time Integrator/1 -> Memory/1
  Memory/1 -> MATLAB Function/7(xi)
  abc to Alpha-Beta-Zero/1 -> Selector4/1
  Selector4/1 -> [ValphaBeta]
  abc to Alpha-Beta-Zero1/1 -> Selector1/1
  Selector1/1 -> [IalphaBeta]
  [ValphaBeta] -> MATLAB Function/8(u_alphabeta)
  [IalphaBeta] -> MATLAB Function/9(i_alphabeta)
  MATLAB Function/2(EMF) -> Scope1/1, [EMF]
  Gain1/1 -> [theta_real]
  [EMF] -> Demux1/1
  Demux1/2 -> Trigonometric Function2/1
  Demux1/1 -> Trigonometric Function2/2
  Constant6/1 -> Math Function2/2, Math Function/2
  [theta_real] -> Math Function/1
  Math Function/1 -> Scope/1
  Trigonometric Function2/1 -> Math Function2/1
  Math Function2/1 -> [thetaE_Est], Scope/2
  [rotor_angle_rad_modi] -> Scope2/2
  [theta_real] -> Scope2/1

== system OberverForPMSM/PMSG Wind Turbine/Control/Crow bar Protection ==
  Vdc_V : Inport
  Relay : Relay  OnSwitchValue=1500  OffSwitchValue=1300
  Pulses_crow_bar : Outport
  wires:
  Vdc_V/1 -> Relay/1
  Relay/1 -> Pulses_crow_bar/1

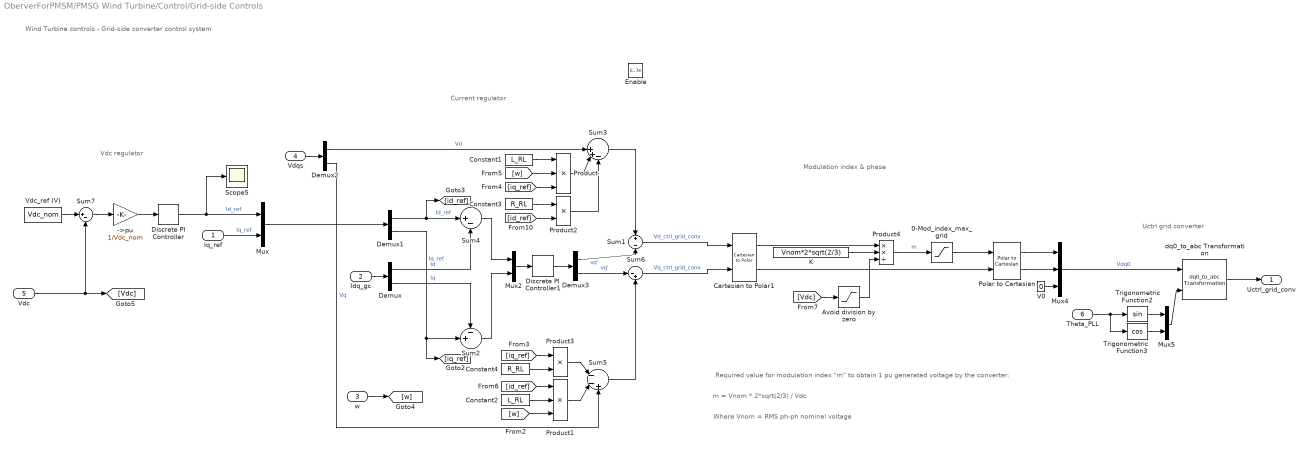
== system OberverForPMSM/PMSG Wind Turbine/Control/Grid-side Controls ==
  note: Wind Turbine controls - Grid-side converter control system
  note: Where Vnom = RMS ph-ph nominal voltage
  note: m = Vnom * 2*sqrt(2/3) / Vdc
  note: Required value for modulation index "m" to obtain 1 pu generated voltage by the converter:
  note: Vdc regulator
  note: Current regulator
  note: Modulation index & phase
  note: Uctrl grid converter
  Iq_ref : Inport
  Idq_gc : Inport  Port=2
  w : Inport  Port=3
  Vdqs : Inport  Port=4
  Vdc : Inport  Port=5
  Theta_PLL : Inport  Port=6
  Enable : EnablePort
  ->pu : Gain  Gain=1/Vdc_nom
  0-Mod_index_max_grid : Saturate  UpperLimit=2  LowerLimit=0
  Avoid division by zero : Saturate  UpperLimit=inf  LowerLimit=1e-6
  Cartesian to Polar1 : simulink_extras/Transformations/Cartesian to Polar
      settings: SourceProductName=Simulink
  Constant1 : Constant  Value=L_RL
  Constant2 : Constant  Value=L_RL
  Constant3 : Constant  Value=R_RL
  Constant4 : Constant  Value=R_RL
  Demux{,1..3} (4 alike) : Demux  Outputs=2
  Discrete PI Controller : powerlib_extras/Discrete  Control Blocks/Discrete PI Controller  Kp=8  Ki=400  Par_Limits=[1 -1]*1.5  Init=-0.5  Ts=Ts
  Discrete PI Controller1 : powerlib_extras/Discrete  Control Blocks/Discrete PI Controller  Kp=0.83  Ki=5  Par_Limits=[1.0 -1.0]*2  Init=0  Ts=Ts
  K : Constant  Value=Vnom*2*sqrt(2/3)
  Mux : Mux  Inputs=2
  Mux2 : Mux  Inputs=2
  Mux4 : Mux  Inputs=3
  Mux5 : Mux  Inputs=2
  Polar to Cartesian : simulink_extras/Transformations/Polar to Cartesian
      settings: SourceProductName=Simulink  SourceProductBaseCode=SL
  Product : Product  Inputs=3  SaturateOnIntegerOverflow=on  InputSameDT=on  OutDataTypeStr=Inherit: Same as first input
  Product1 : Product  Inputs=3  SaturateOnIntegerOverflow=on  InputSameDT=on  OutDataTypeStr=Inherit: Same as first input
  Product2 : Product  SaturateOnIntegerOverflow=on  InputSameDT=on  OutDataTypeStr=Inherit: Same as first input
  Product3 : Product  SaturateOnIntegerOverflow=on  InputSameDT=on  OutDataTypeStr=Inherit: Same as first input
  Product4 : Product  Inputs=**/  SaturateOnIntegerOverflow=on  InputSameDT=on  OutDataTypeStr=Inherit: Same as first input
  Scope5 : Scope
  Sum1 : Sum  Inputs=+-  SaturateOnIntegerOverflow=on  InputSameDT=on  OutDataTypeStr=Inherit: Same as first input
  Sum2 : Sum  Inputs=-+|  SaturateOnIntegerOverflow=on  InputSameDT=on  OutDataTypeStr=Inherit: Same as first input
  Sum3 : Sum  Inputs=||++-  SaturateOnIntegerOverflow=on  InputSameDT=on  OutDataTypeStr=Inherit: Same as first input
  Sum4 : Sum  Inputs=|+-  SaturateOnIntegerOverflow=on  InputSameDT=on  OutDataTypeStr=Inherit: Same as first input
  Sum5 : Sum  Inputs=|--+  SaturateOnIntegerOverflow=on  InputSameDT=on  OutDataTypeStr=Inherit: Same as first input
  Sum6 : Sum  Inputs=|-+  SaturateOnIntegerOverflow=on  InputSameDT=on  OutDataTypeStr=Inherit: Same as first input
  Sum7 : Sum  Inputs=|+-  SaturateOnIntegerOverflow=on  InputSameDT=on  OutDataTypeStr=Inherit: Same as first input
  Trigonometric Function2 : Trigonometry
  Trigonometric Function3 : Trigonometry  Operator=cos
  V0 : Constant  Value=0
  Vdc_ref (V) : Constant  Value=Vdc_nom
  dq0_to_abc Transformation : powerlib_extras/Measurements/dq0_to_abc Transformation
  Uctrl_grid_conv : Outport
  wires:
  Vdc_ref (V)/1 -> Sum7/1
  Iq_ref/1 -> Mux/2  "Iq_ref"
  ->pu/1 -> Discrete PI Controller/1
  Sum7/1 -> ->pu/1
  Discrete PI Controller/1 -> Mux/1, Scope5/1  "Id_ref"
  Sum5/1 -> Sum6/2
  Sum3/1 -> Sum1/1
  Demux1/1 -> [id_ref], Sum4/1  "Id_ref"
  Demux1/2 -> Sum2/2, [iq_ref]  "Iq_ref"
  Demux3/2 -> Sum6/1  "vq'"
  Demux3/1 -> Sum1/2  "vd'"
  [id_ref] -> Product1/1
  [iq_ref] -> Product3/1
  [id_ref] -> Product2/2
  [iq_ref] -> Product/3
  [w] -> Product/2
  [w] -> Product1/3
  Sum2/1 -> Mux2/2
  Sum4/1 -> Mux2/1
  Product3/1 -> Sum5/1
  Product2/1 -> Sum3/3
  Demux2/2 -> Sum5/3  "Vq"
  Product1/1 -> Sum5/2
  Constant4/1 -> Product3/2
  Constant3/1 -> Product2/1
  Product/1 -> Sum3/2
  Vdqs/1 -> Demux2/1
  Constant1/1 -> Product/1
  Demux2/1 -> Sum3/1  "Vd"
  Mux2/1 -> Discrete PI Controller1/1
  Discrete PI Controller1/1 -> Demux3/1
  Constant2/1 -> Product1/2
  w/1 -> [w]
  Mux/1 -> Demux1/1
  Cartesian to Polar1/2 -> Polar to Cartesian/2
  0-Mod_index_max_grid/1 -> Polar to Cartesian/1
  Cartesian to Polar1/1 -> Product4/1
  Avoid division by zero/1 -> Product4/3
  K/1 -> Product4/2
  Product4/1 -> 0-Mod_index_max_grid/1  "m"
  [Vdc] -> Avoid division by zero/1
  Mux5/1 -> dq0_to_abc Transformation/2
  Trigonometric Function2/1 -> Mux5/1
  Trigonometric Function3/1 -> Mux5/2
  V0/1 -> Mux4/3
  Polar to Cartesian/1 -> Mux4/1
  Polar to Cartesian/2 -> Mux4/2
  Mux4/1 -> dq0_to_abc Transformation/1  "Vdq0"
  Theta_PLL/1 -> Trigonometric Function3/1, Trigonometric Function2/1
  dq0_to_abc Transformation/1 -> Uctrl_grid_conv/1
  Sum1/1 -> Cartesian to Polar1/1  "Vd_ctrl_grid_conv"
  Sum6/1 -> Cartesian to Polar1/2  "Vq_ctrl_grid_conv"
  Vdc/1 -> Sum7/2, [Vdc]
  Idq_gc/1 -> Demux/1
  Demux/1 -> Sum4/2  "Id"
  Demux/2 -> Sum2/1  "Iq"

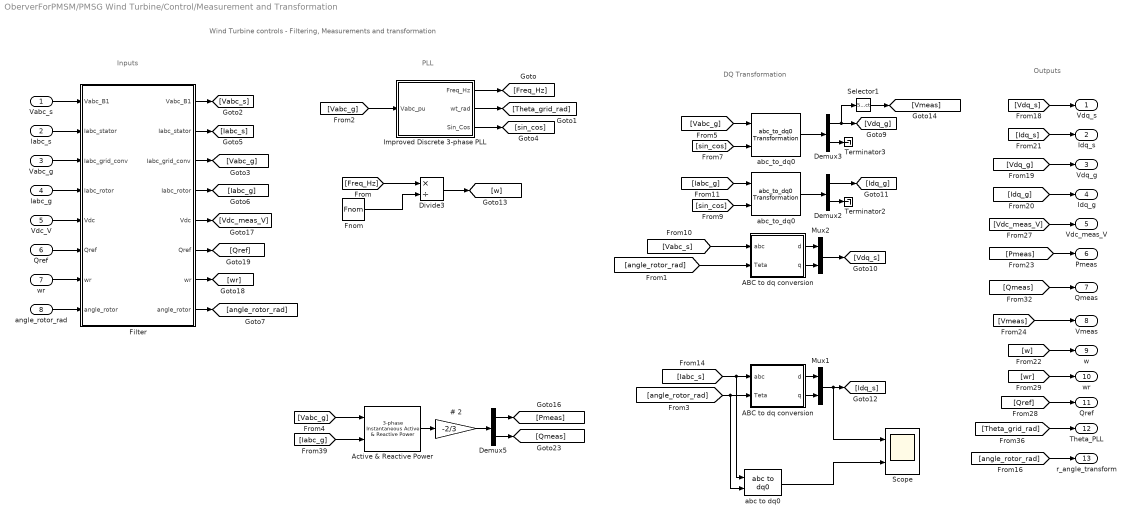
== system OberverForPMSM/PMSG Wind Turbine/Control/Measurement and Transformation ==
  note: Wind Turbine controls - Filtering, Measurements and transformation
  note: Outputs
  note: Inputs
  note: PLL
  note: DQ Transformation
  Vabc_s : Inport
  Iabc_s : Inport  Port=2
  Vabc_g : Inport  Port=3
  Iabc_g : Inport  Port=4
  Vdc_V : Inport  Port=5
  Qref : Inport  Port=6
  wr : Inport  Port=7
  angle_rotor_rad : Inport  Port=8
  " Improved Discrete 3-phase PLL" : Subsystem  AncestorBlock=|  mask(Discrete 3-phase PLL){Fmin=0.75*Fnom, Par_Init=[0 Fnom], ParK=[5 3.2 1 50], Ts=Ts}
      | powerlib_extras/Discrete 
      | Control Blocks/Discrete
      | 3-phase PLL
      mask prompts: Fmin "Minimum frequency (Hz):"; Par_Init "Initial inputs:[ Phase(degrees)   Frequency(Hz) ]"; ParK "Regulator gains [ Kp1 Kp2  Ki1  Ki2 ]"; Ts "Sample time:"
      mask help:
      | This Phase Locked Loop (PLL) system can be used  to synchronize on a set of variable frequency, three-phase sinusoidal signals.
      |
      | Input 1: Vector containing the normalized
      |              three-phase signals [Va Vb Vc]
      | Output 1:  Measured frequency (Hz) = w/(2pi)
      | Output 2:  Ramp w.t   varying between  0 and 2*pi,
      | synchronized on zero crossings of the fundamental (positive-sequence) of phase A.
      | Output 3: Vector [sin(wt) cos(wt)]
      mask init:
      | Kp1=ParK(1);
      | Kp2=ParK(2);
      | Ki1=ParK(3);
      | Ki2=ParK(4);
      | Phase_Init=Par_Init(1);
      | Finit=Par_Init(2);
      | power_initmask();
      settings: OpenFcn=power_openblockproxy();
  # 2 : Gain  Gain=-2/3  SaturateOnIntegerOverflow=on  OutDataTypeStr=Inherit: Same as input  ParamDataTypeStr=Inherit: Same as input
  "ABC to dq conversion " : Subsystem
  ABC to dq conversion : Subsystem
  Active & Reactive Power : powerlib_extras/Measurements/3-phase  Instantaneous  Active & Reactive Power
  Demux2 : Demux  Outputs=[2 1]
  Demux3 : Demux  Outputs=[2 1]
  Demux5 : Demux  Outputs=2
  Divide3 : Product  Inputs=*/
  Filter : Subsystem  mask{Freq=1e4, Zeta1=0.707, Ts=Ts}
      mask prompts: Freq "Cut-off frequency (Hz):"; Zeta1 "Damping factor Zeta:"; Ts "Sample time"
  Fnom : Constant  Value=Fnom
  Mux1 : Mux  Inputs=2
  Mux2 : Mux  Inputs=2
  Scope : Scope  NumInputPorts=2
  Selector1 : Selector  InputPortWidth=2  IndexOptions=Index vector (dialog)  Indices=1  OutputSizes=[(-2)]
  Terminator2 : Terminator
  Terminator3 : Terminator
  abc to dq0 : powerlib_meascontrol/Transformations/abc to dq0  Alignment=Aligned with phase A axis
  abc_to_dq0 : powerlib_extras/Measurements/abc_to_dq0 Transformation
  "abc_to_dq0 " : powerlib_extras/Measurements/abc_to_dq0 Transformation
  Vdq_s : Outport
  Idq_s : Outport  Port=2
  Vdq_g : Outport  Port=3
  Idq_g : Outport  Port=4
  Vdc_meas_V : Outport  Port=5
  Pmeas : Outport  Port=6
  Qmeas : Outport  Port=7
  Vmeas : Outport  Port=8
  w : Outport  Port=9
  "wr " : Outport  Port=10
  "Qref " : Outport  Port=11
  Theta_PLL : Outport  Port=12
  r_angle_transform : Outport  Port=13
  wires:
  angle_rotor_rad/1 -> Filter/8(angle_rotor)
  Filter/8("angle_rotor ") -> [angle_rotor_rad]
  Filter/7("wr ") -> [wr]
  Filter/6("Qref ") -> [Qref]
  Filter/5("Vdc ") -> [Vdc_meas_V]
  Filter/4("Iabc_rotor ") -> [Iabc_g]
  Filter/3("Iabc_grid_conv ") -> [Vabc_g]
  Filter/2("Iabc_stator ") -> [Iabc_s]
  Filter/1("Vabc_B1 ") -> [Vabc_s]
  [wr] -> "wr "/1
  [Qref] -> "Qref "/1
  [Vdc_meas_V] -> Vdc_meas_V/1
  wr/1 -> Filter/7(wr)
  Qref/1 -> Filter/6(Qref)
  Vdc_V/1 -> Filter/5(Vdc)
  Iabc_g/1 -> Filter/4(Iabc_rotor)
  Vabc_g/1 -> Filter/3(Iabc_grid_conv)
  Iabc_s/1 -> Filter/2(Iabc_stator)
  Vabc_s/1 -> Filter/1(Vabc_B1)
  [angle_rotor_rad] -> abc to dq0/2, "ABC to dq conversion "/2(Teta)
  [Vmeas] -> Vmeas/1
  [Pmeas] -> Pmeas/1
  [w] -> w/1
  [Idq_s] -> Idq_s/1
  [Idq_g] -> Idq_g/1
  [Vdq_g] -> Vdq_g/1
  [Vdq_s] -> Vdq_s/1
  Demux2/1 -> [Idq_g]
  [Iabc_s] -> abc to dq0/1, "ABC to dq conversion "/1(abc)
  [Iabc_g] -> "abc_to_dq0 "/1
  [Vabc_s] -> ABC to dq conversion/1(abc)
  [sin_cos] -> "abc_to_dq0 "/2
  [sin_cos] -> abc_to_dq0/2
  [Vabc_g] -> abc_to_dq0/1
  [Freq_Hz] -> Divide3/1
  Divide3/1 -> [w]
  Fnom/1 -> Divide3/2
  "abc_to_dq0 "/1 -> Demux2/1
  Demux2/2 -> Terminator2/1
  abc_to_dq0/1 -> Demux3/1
  Demux3/2 -> Terminator3/1
  Demux3/1 -> [Vdq_g], Selector1/1
  [Qmeas] -> Qmeas/1
  [Theta_grid_rad] -> Theta_PLL/1
  [angle_rotor_rad] -> r_angle_transform/1
  [Vabc_g] -> " Improved Discrete 3-phase PLL"/1(Vabc_pu)
  " Improved Discrete 3-phase PLL"/2(wt_rad) -> [Theta_grid_rad]
  " Improved Discrete 3-phase PLL"/3(Sin_Cos) -> [sin_cos]
  " Improved Discrete 3-phase PLL"/1(Freq_Hz) -> [Freq_Hz]
  [Vabc_g] -> Active & Reactive Power/1
  [Iabc_g] -> Active & Reactive Power/2
  Demux5/1 -> [Pmeas]
  Demux5/2 -> [Qmeas]
  Active & Reactive Power/1 -> # 2/1
  # 2/1 -> Demux5/1
  Selector1/1 -> [Vmeas]
  [angle_rotor_rad] -> ABC to dq conversion/2(Teta)
  ABC to dq conversion/1(d) -> Mux2/1
  ABC to dq conversion/2(q) -> Mux2/2
  Mux2/1 -> [Vdq_s]
  "ABC to dq conversion "/1(d) -> Mux1/1
  "ABC to dq conversion "/2(q) -> Mux1/2
  Mux1/1 -> Scope/1, [Idq_s]
  abc to dq0/1 -> Scope/2

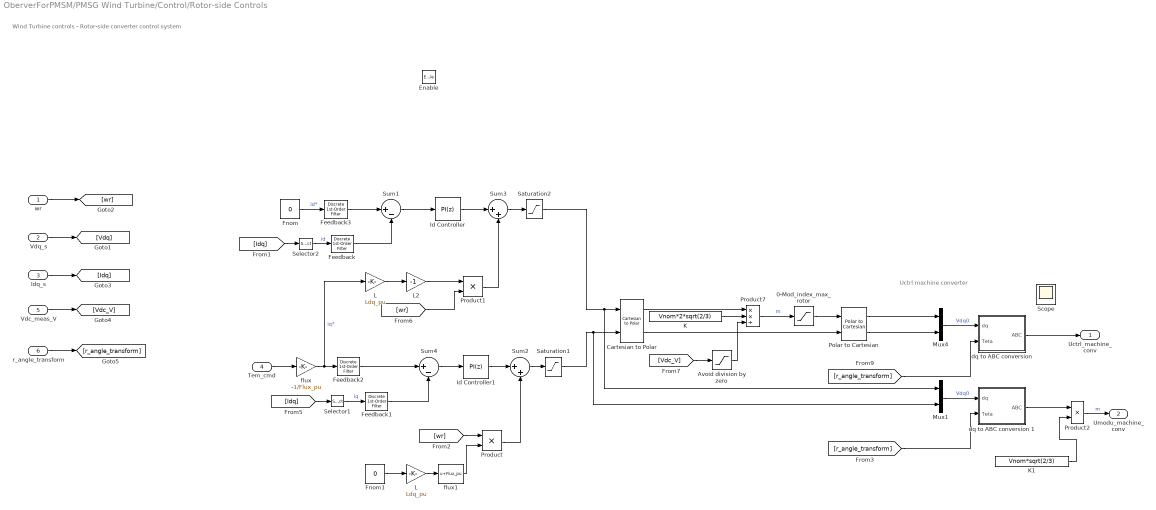
== system OberverForPMSM/PMSG Wind Turbine/Control/Rotor-side Controls ==
  note: Wind Turbine controls - Rotor-side converter control system
  note: Uctrl machine converter
  wr : Inport
  " Vdq_s" : Inport  Port=2
  Idq_s : Inport  Port=3
  Tem_cmd : Inport  Port=4
  Vdc_meas_V : Inport  Port=5
  r_angle_transform : Inport  Port=6
  Enable : EnablePort
  0-Mod_index_max_rotor : Saturate  UpperLimit=2  LowerLimit=0
  Avoid division by zero : Saturate  UpperLimit=inf  LowerLimit=1e-6
  Cartesian to Polar : simulink_extras/Transformations/Cartesian to Polar
      settings: SourceProductName=Simulink
  Feedback : powerlib_extras/Discrete  Control Blocks/Discrete 1st-Order Filter  FilterType=Lowpass  Tc=Fb_time_const  Ts=Ts  Initialize=on  Vac_Init=[0 -25 60]  Vdc_Init=0  PlotResponse=off  param1=[1 500 0.1]
  Feedback1 : powerlib_extras/Discrete  Control Blocks/Discrete 1st-Order Filter  FilterType=Lowpass  Tc=Fb_time_const  Ts=Ts  Initialize=on  Vac_Init=[0 -25 60]  Vdc_Init=0  PlotResponse=off  param1=[1 500 0.1]
  Feedback2 : powerlib_extras/Discrete  Control Blocks/Discrete 1st-Order Filter  FilterType=Lowpass  Tc=Fb_time_const  Ts=Ts  Initialize=on  Vac_Init=[0 -25 60]  Vdc_Init=0.5  PlotResponse=off  param1=[1 500 0.1]
  Feedback3 : powerlib_extras/Discrete  Control Blocks/Discrete 1st-Order Filter  FilterType=Lowpass  Tc=Fb_time_const  Ts=Ts  Initialize=on  Vac_Init=[0 -25 60]  Vdc_Init=0  PlotResponse=off  param1=[1 500 0.1]
  Fnom : Constant  Value=0
  Fnom1 : Constant  Value=0
  Id Controller : simulink/Continuous/PID Controller  Controller=PI  Form=Parallel  TimeDomain=Discrete-time  SampleTime=Ts  IntegratorMethod=Forward Euler  FilterMethod=Forward Euler  ControllerParametersSource=internal  P=0.03*2129.991/469.486  I=(0.03/0.05)*2129.991/469.486  D=0  UseFilter=on  N=100  TunerSelectOption=Transfer Function Based (PID Tuner App)  ZeroCross=off  InitialConditionSource=internal  InitialConditionForIntegrator=0  InitialConditionForFilter=0  DifferentiatorICPrevScaledInput=0  ExternalReset=none  TrackingMode=off  Kt=1  LimitOutput=on  UpperSaturationLimit=5  LowerSaturationLimit=-5  LinearizeAsGain=off  AntiWindupMode=clamping  Kb=1  POutMin=[]  POutMax=[]  IOutMin=[]  IOutMax=[]  DOutMin=[]  DOutMax=[]  NOutMin=[]  NOutMax=[]  SumOutMin=[]  SumOutMax=[]  SaturationOutMin=[]  SaturationOutMax=[]  PParamMin=[]  PParamMax=[]  IParamMin=[]  IParamMax=[]  DParamMin=[]  DParamMax=[]  NParamMin=[]  NParamMax=[]  KbParamMin=[]  KbParamMax=[]  KtParamMin=[]  KtParamMax=[]  KbOutMin=[]  KbOutMax=[]  KtOutMin=[]  KtOutMax=[]  IntegratorOutMin=[]  IntegratorOutMax=[]  FilterOutMin=[]  FilterOutMax=[]  SumI1OutMin=[]  SumI1OutMax=[]  SumI2OutMin=[]  SumI2OutMax=[]  SumI3OutMin=[]  SumI3OutMax=[]  SumI4OutMin=[]  SumI4OutMax=[]  SumDOutMin=[]  SumDOutMax=[]  DifferentiatorOutMin=[]  DifferentiatorOutMax=[]  FilterDiffOutCoefMin=[]  FilterDiffOutCoefMax=[]  ReciprocalOutMin=[]  ReciprocalOutMax=[]  SumDenOutMin=[]  SumDenOutMax=[]  SumNumOutMin=[]  SumNumOutMax=[]  DivideOutMin=[]  DivideOutMax=[]  IntegratorContinuousStateAttributes=''  IntegratorStateMustResolveToSignalObject=off  IntegratorRTWStateStorageClass=Auto  FilterContinuousStateAttributes=''  FilterStateMustResolveToSignalObject=off  FilterRTWStateStorageClass=Auto  ParallelPVariant=InternalParameters  IdealPVariant=Disabled  IVariant=InternalParameters  DVariant=Disabled  IntegratorVariant=Discrete  SatVariant=Enabled  AWVariant=DiscClampingParallel  PCopyVariant=Disabled  TRVariant=Disabled  FdbkBlocksVariant=Forward  IdealPFdbkVariant=Disabled  SatFdbkVariant=Disabled  DerivativeFilterVariant=Disabled  NVariant=Disabled  NCopyVariant=Disabled_SignalSpec  FilterICVariant=Disabled  IntegratorICVariant=InternalICs  ExternalResetVariant=Disabled  TRSumVariant=Passthrough  SumFdbkVariant=Disabled  SumVariant=Sum_PI
  Id Controller1 : simulink/Continuous/PID Controller  Controller=PI  Form=Parallel  TimeDomain=Discrete-time  SampleTime=Ts  IntegratorMethod=Forward Euler  FilterMethod=Forward Euler  ControllerParametersSource=internal  P=0.03*2129.991/469.486  I=(0.03/0.05)*2129.991/469.486  D=0  UseFilter=on  N=100  TunerSelectOption=Transfer Function Based (PID Tuner App)  ZeroCross=off  InitialConditionSource=internal  InitialConditionForIntegrator=0  InitialConditionForFilter=0  DifferentiatorICPrevScaledInput=0  ExternalReset=none  TrackingMode=off  Kt=1  LimitOutput=on  UpperSaturationLimit=5  LowerSaturationLimit=-5  LinearizeAsGain=off  AntiWindupMode=clamping  Kb=1  POutMin=[]  POutMax=[]  IOutMin=[]  IOutMax=[]  DOutMin=[]  DOutMax=[]  NOutMin=[]  NOutMax=[]  SumOutMin=[]  SumOutMax=[]  SaturationOutMin=[]  SaturationOutMax=[]  PParamMin=[]  PParamMax=[]  IParamMin=[]  IParamMax=[]  DParamMin=[]  DParamMax=[]  NParamMin=[]  NParamMax=[]  KbParamMin=[]  KbParamMax=[]  KtParamMin=[]  KtParamMax=[]  KbOutMin=[]  KbOutMax=[]  KtOutMin=[]  KtOutMax=[]  IntegratorOutMin=[]  IntegratorOutMax=[]  FilterOutMin=[]  FilterOutMax=[]  SumI1OutMin=[]  SumI1OutMax=[]  SumI2OutMin=[]  SumI2OutMax=[]  SumI3OutMin=[]  SumI3OutMax=[]  SumI4OutMin=[]  SumI4OutMax=[]  SumDOutMin=[]  SumDOutMax=[]  DifferentiatorOutMin=[]  DifferentiatorOutMax=[]  FilterDiffOutCoefMin=[]  FilterDiffOutCoefMax=[]  ReciprocalOutMin=[]  ReciprocalOutMax=[]  SumDenOutMin=[]  SumDenOutMax=[]  SumNumOutMin=[]  SumNumOutMax=[]  DivideOutMin=[]  DivideOutMax=[]  IntegratorContinuousStateAttributes=''  IntegratorStateMustResolveToSignalObject=off  IntegratorRTWStateStorageClass=Auto  FilterContinuousStateAttributes=''  FilterStateMustResolveToSignalObject=off  FilterRTWStateStorageClass=Auto  ParallelPVariant=InternalParameters  IdealPVariant=Disabled  IVariant=InternalParameters  DVariant=Disabled  IntegratorVariant=Discrete  SatVariant=Enabled  AWVariant=DiscClampingParallel  PCopyVariant=Disabled  TRVariant=Disabled  FdbkBlocksVariant=Forward  IdealPFdbkVariant=Disabled  SatFdbkVariant=Disabled  DerivativeFilterVariant=Disabled  NVariant=Disabled  NCopyVariant=Disabled_SignalSpec  FilterICVariant=Disabled  IntegratorICVariant=InternalICs  ExternalResetVariant=Disabled  TRSumVariant=Passthrough  SumFdbkVariant=Disabled  SumVariant=Sum_PI
  K : Constant  Value=Vnom*2*sqrt(2/3)
  K1 : Constant  Value=Vnom*sqrt(2/3)
  L : Gain  Gain=Ldq_pu
  "L  " : Gain  Gain=Ldq_pu
  L2 : Gain  Gain=-1
  Mux1 : Mux  Inputs=2
  Mux4 : Mux  Inputs=2
  Polar to Cartesian : simulink_extras/Transformations/Polar to Cartesian
      settings: SourceProductName=Simulink  SourceProductBaseCode=SL
  Product : Product  RndMeth=Zero
  Product1 : Product  RndMeth=Zero
  Product2 : Product  Inputs=**  SaturateOnIntegerOverflow=on  InputSameDT=on  OutDataTypeStr=Inherit: Same as first input
  Product7 : Product  Inputs=**/  SaturateOnIntegerOverflow=on  InputSameDT=on  OutDataTypeStr=Inherit: Same as first input
  Saturation1 : Saturate  UpperLimit=5  LowerLimit=-5  SampleTime=Ts
  Saturation2 : Saturate  UpperLimit=5  LowerLimit=-5  SampleTime=Ts
  Scope : Scope
  Selector1 : Selector  InputPortWidth=2  IndexOptions=Index vector (dialog)  Indices=2  OutputSizes=[(-2)]
  Selector2 : Selector  InputPortWidth=2  IndexOptions=Index vector (dialog)  Indices=1  OutputSizes=[(-2)]
  Sum1 : Sum  Inputs=|+-  SaturateOnIntegerOverflow=on  InputSameDT=on  OutDataTypeStr=Inherit: Same as first input
  Sum2 : Sum  Inputs=|++  SaturateOnIntegerOverflow=on  InputSameDT=on  OutDataTypeStr=Inherit: Same as first input
  Sum3 : Sum  Inputs=|++  SaturateOnIntegerOverflow=on  InputSameDT=on  OutDataTypeStr=Inherit: Same as first input
  Sum4 : Sum  Inputs=|+-  SaturateOnIntegerOverflow=on  InputSameDT=on  OutDataTypeStr=Inherit: Same as first input
  "dq to ABC conversion " : Subsystem
  dq to ABC conversion 1 : Subsystem
  flux : Gain  Gain=-1/Flux_pu
  flux1 : Bias  Bias=Flux_pu
  Uctrl_machine_conv : Outport
  Umodu_machine_conv : Outport  Port=2
  wires:
  Tem_cmd/1 -> flux/1
  wr/1 -> [wr]
  " Vdq_s"/1 -> [Vdq]
  Idq_s/1 -> [Idq]
  Vdc_meas_V/1 -> [Vdc_V]
  r_angle_transform/1 -> [r_angle_transform]
  [Idq] -> Selector1/1
  Sum4/1 -> Id Controller1/1
  [Idq] -> Selector2/1
  Sum1/1 -> Id Controller/1
  Id Controller1/1 -> Sum2/1
  Id Controller/1 -> Sum3/1
  [wr] -> Product/1
  flux1/1 -> Product/2
  L/1 -> flux1/1
  "L  "/1 -> L2/1
  L2/1 -> Product1/1
  [wr] -> Product1/2
  Cartesian to Polar/1 -> Product7/1
  K/1 -> Product7/2
  Mux4/1 -> "dq to ABC conversion "/1(dq)  "Vdq0"
  Avoid division by zero/1 -> Product7/3
  [Vdc_V] -> Avoid division by zero/1
  Product7/1 -> 0-Mod_index_max_rotor/1  "m"
  Cartesian to Polar/2 -> Polar to Cartesian/2
  0-Mod_index_max_rotor/1 -> Polar to Cartesian/1
  Polar to Cartesian/1 -> Mux4/1
  Polar to Cartesian/2 -> Mux4/2
  Selector2/1 -> Feedback/1  "id"
  Feedback/1 -> Sum1/2
  Feedback1/1 -> Sum4/2
  Product1/1 -> Sum3/2
  Product/1 -> Sum2/2
  Selector1/1 -> Feedback1/1  "iq"
  [r_angle_transform] -> "dq to ABC conversion "/2(Teta)
  "dq to ABC conversion "/1(ABC) -> Uctrl_machine_conv/1
  Sum3/1 -> Saturation2/1
  Saturation2/1 -> Mux1/1, Cartesian to Polar/1
  Sum2/1 -> Saturation1/1
  Saturation1/1 -> Mux1/2, Cartesian to Polar/2
  flux/1 -> Feedback2/1, "L  "/1  "iq*"
  Feedback2/1 -> Sum4/1
  Feedback3/1 -> Sum1/1
  Fnom/1 -> Feedback3/1  "id*"
  Fnom1/1 -> L/1
  [r_angle_transform] -> dq to ABC conversion 1/2(Teta)
  Mux1/1 -> dq to ABC conversion 1/1(dq)  "Vdq0"
  dq to ABC conversion 1/1(ABC) -> Product2/1
  Product2/1 -> Umodu_machine_conv/1  "m"
  K1/1 -> Product2/2
